simulink model "thread_id_calc"  (Simulink 7.7)
settings: Solver=ode45  StartTime=0.0  StopTime=100.0  RelTol=1e-3
undefined symbols (not defined in the file): xlipgetpartsetting
libraries: xbsIndex_r4 x50
settings Model: Creator=Andryc  LastModifiedBy=andryc

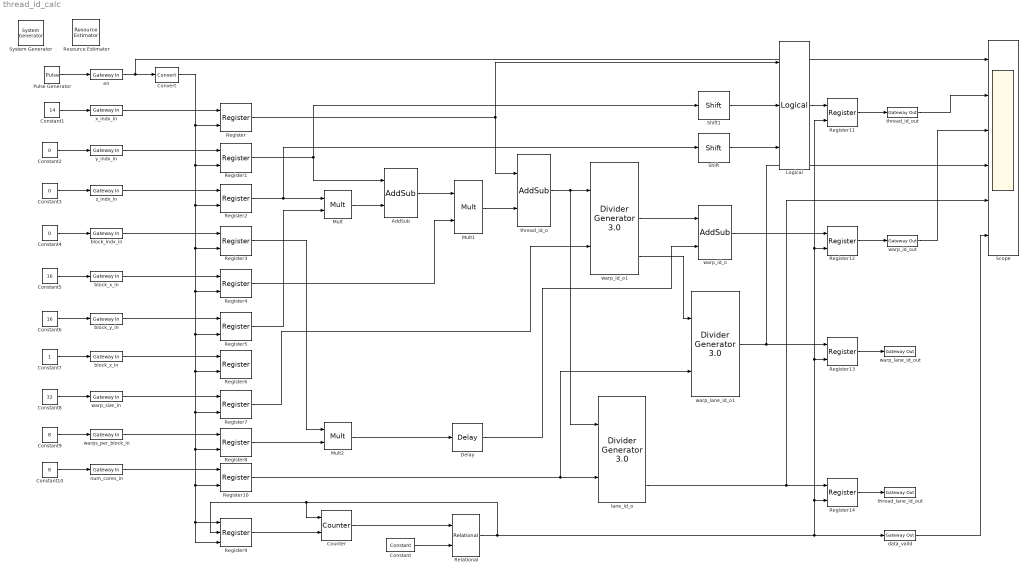
== system thread_id_calc ==
  " System Generator" : xbsIndex_r4/ System Generator  Tag=genX  SystemSampleTime=-1  xilinxfamily=virtex6  part=xc6vlx240t  speed=-2  package=ff1156  synthesis_tool=XST  clock_wrapper=Clock Enables  directory=./netlist  proj_type=Project Navigator  Synth_file=XST Defaults  Impl_file=ISE Defaults  testbench=on  simulink_period=1  sysclk_period=10  dcm_input_clock_period=10  incr_netlist=off  trim_vbits=Everywhere in SubSystem  dbl_ovrd=According to Block Masks  core_generation=According to Block Masks  run_coregen=off  deprecated_control=off  eval_field=0  block_type=sysgen
  AddSub : xbsIndex_r4/AddSub  mode=Addition  use_carryin=off  use_carryout=off  en=off  latency=0  precision=User Defined  arith_type=Unsigned  n_bits=32  bin_pt=0  quantization=Truncate  overflow=Saturate  dbl_ovrd=off  use_behavioral_HDL=off  hw_selection=Fabric  pipelined=off  block_type=addsub
  Constant : xbsIndex_r4/Constant  const=48  gui_display_data_type=Fixed-point  arith_type=Unsigned  n_bits=8  bin_pt=0  preci_type=Single  exp_width=8  frac_width=24  explicit_period=off  period=1  equ=P=C  opselect=C  inp2=PCIN>>17  opr=+  inp1=P  carry=CIN  dbl_ovrd=off  block_type=constant
  Constant1 : Constant  Value=14
  Constant10 : Constant  Value=8
  Constant2 : Constant  Value=0
  Constant3 : Constant  Value=0
  Constant4 : Constant  Value=0
  Constant5 : Constant  Value=16
  Constant6 : Constant  Value=16
  Constant7 : Constant
  Constant8 : Constant  Value=32
  Constant9 : Constant  Value=8
  Convert : xbsIndex_r4/Convert  gui_display_data_type=Boolean  arith_type=Boolean  n_bits=16  bin_pt=14  float_type=Single  exp_bits=8  fraction_bits=24  quantization=Truncate  overflow=Wrap  en=off  latency=0  dbl_ovrd=off  pipeline=off  block_type=convert
  Counter : xbsIndex_r4/Counter  cnt_type=Free Running  cnt_to=Inf  operation=Up  start_count=0  cnt_by_val=1  arith_type=Unsigned  n_bits=8  bin_pt=0  load_pin=off  rst=on  en=on  explicit_period=on  period=1  dbl_ovrd=off  use_behavioral_HDL=off  implementation=Fabric  block_type=counter
  Delay : xbsIndex_r4/Delay  rst=off  infoeditControl=Selection of Reset will increase slice count due to use of real FFs and instead of SRLs  en=off  latency=3  dbl_ovrd=off  reg_retiming=off  block_type=delay
  Logical : xbsIndex_r4/Logical  logical_function=OR  inputs=3  en=off  latency=0  precision=User Defined  arith_type=Unsigned  n_bits=32  bin_pt=0  align_bp=on  dbl_ovrd=off  block_type=logical
  Mult : xbsIndex_r4/Mult  precision=User Defined  arith_type=Unsigned  n_bits=32  bin_pt=0  quantization=Truncate  overflow=Saturate  en=off  latency=3  dbl_ovrd=off  use_behavioral_HDL=off  opt=Speed  use_embedded=on  optimum_pipeline=off  pipeline=on  use_rpm=on  placement_style=Triangular  block_type=mult
  Mult1 : xbsIndex_r4/Mult  precision=User Defined  arith_type=Unsigned  n_bits=32  bin_pt=0  quantization=Truncate  overflow=Saturate  en=off  latency=3  dbl_ovrd=off  use_behavioral_HDL=off  opt=Speed  use_embedded=on  optimum_pipeline=off  pipeline=on  use_rpm=on  placement_style=Triangular  block_type=mult
  Mult2 : xbsIndex_r4/Mult  precision=Full  arith_type="Signed  (2's comp)"  n_bits=16  bin_pt=14  quantization=Truncate  overflow=Wrap  en=off  latency=3  dbl_ovrd=off  use_behavioral_HDL=off  opt=Speed  use_embedded=on  optimum_pipeline=off  pipeline=on  use_rpm=on  placement_style=Triangular  block_type=mult
  Pulse Generator : DiscretePulseGenerator  Period=100  PhaseDelay=10
  Register{,1..8,10..14} (14 alike) : xbsIndex_r4/Register  init=0  rst=off  en=on  dbl_ovrd=off  block_type=register
  Register9 : xbsIndex_r4/Register  init=0  rst=on  en=on  dbl_ovrd=off  block_type=register
  Relational : xbsIndex_r4/Relational  mode=a=b  en=off  latency=0  dbl_ovrd=off  block_type=relational
  Resource Estimator : xbsIndex_r4/Resource Estimator  Tag=resEstTag  Slices=0  FFs=0  BRAMs=0  LUTs=0  IOBs=0  EBMs=0  TBUFs=0  xl_use_estimator_area=off  est_options=Estimate  block_type=resource_estimator
      settings: AttributesFormatString=Resource\nEstimator
  Scope : Scope  NumInputPorts=6
      settings: YMin=-5~-5~-5~-5~-5~-5  YMax=5~5~5~5~5~5
  Shift : xbsIndex_r4/Shift  shift_dir=Left  shift_bits=26  en=off  latency=0  precision=User Defined  arith_type=Unsigned  n_bits=32  bin_pt=0  quantization=Truncate  overflow=Saturate  dbl_ovrd=off  block_type=shift
  Shift1 : xbsIndex_r4/Shift  shift_dir=Left  shift_bits=16  en=off  latency=0  precision=User Defined  arith_type=Unsigned  n_bits=32  bin_pt=0  quantization=Truncate  overflow=Saturate  dbl_ovrd=off  block_type=shift
  block_indx_in : xbsIndex_r4/Gateway In  gui_display_data_type=Fixed-point  arith_type=Unsigned  n_bits=16  bin_pt=0  preci_type=Single  exp_width=8  frac_width=24  quantization=Truncate  overflow=Saturate  period=1  dbl_ovrd=off  timing_constraint=None  locs_specified=off  LOCs={}  inherit_from_input=off  UseAsADC=off  ADCChannel='1'  hdl_port=on  block_type=gatewayin
      settings: infoedit="Gateway in block.  Converts inputs of type Simulink integer, single, double and fixed point to  Xilinx fixed-point or floating-point data type.<br><br>Hardware notes:  In hardware these blocks become top level input ports."
  block_x_in : xbsIndex_r4/Gateway In  gui_display_data_type=Fixed-point  arith_type=Unsigned  n_bits=16  bin_pt=0  preci_type=Single  exp_width=8  frac_width=24  quantization=Truncate  overflow=Saturate  period=1  dbl_ovrd=off  timing_constraint=None  locs_specified=off  LOCs={}  inherit_from_input=off  UseAsADC=off  ADCChannel='1'  hdl_port=on  block_type=gatewayin
      settings: infoedit="Gateway in block.  Converts inputs of type Simulink integer, single, double and fixed point to  Xilinx fixed-point or floating-point data type.<br><br>Hardware notes:  In hardware these blocks become top level input ports."
  block_y_in : xbsIndex_r4/Gateway In  gui_display_data_type=Fixed-point  arith_type=Unsigned  n_bits=16  bin_pt=0  preci_type=Single  exp_width=8  frac_width=24  quantization=Truncate  overflow=Saturate  period=1  dbl_ovrd=off  timing_constraint=None  locs_specified=off  LOCs={}  inherit_from_input=off  UseAsADC=off  ADCChannel='1'  hdl_port=on  block_type=gatewayin
      settings: infoedit="Gateway in block.  Converts inputs of type Simulink integer, single, double and fixed point to  Xilinx fixed-point or floating-point data type.<br><br>Hardware notes:  In hardware these blocks become top level input ports."
  block_z_in : xbsIndex_r4/Gateway In  gui_display_data_type=Fixed-point  arith_type=Unsigned  n_bits=16  bin_pt=0  preci_type=Single  exp_width=8  frac_width=24  quantization=Truncate  overflow=Saturate  period=1  dbl_ovrd=off  timing_constraint=None  locs_specified=off  LOCs={}  inherit_from_input=off  UseAsADC=off  ADCChannel='1'  hdl_port=on  block_type=gatewayin
      settings: infoedit="Gateway in block.  Converts inputs of type Simulink integer, single, double and fixed point to  Xilinx fixed-point or floating-point data type.<br><br>Hardware notes:  In hardware these blocks become top level input ports."
  data_valid : xbsIndex_r4/Gateway Out  inherit_from_input=off  hdl_port=on  timing_constraint=None  locs_specified=off  LOCs={}  UseAsDAC=off  DACChannel='1'  block_type=gatewayout
      settings: infoedit="Gateway out block.  Converts Xilinx fixed-point or floating-point type inputs into ouputs of type Simulink integer, single, double, or fixed point.<br><br>Hardware notes:  In hardware these blocks become top level output ports or are discarded, depending on how they are configured."
  en : xbsIndex_r4/Gateway In  gui_display_data_type=Fixed-point  arith_type=Unsigned  n_bits=1  bin_pt=0  preci_type=Single  exp_width=8  frac_width=24  quantization=Truncate  overflow=Saturate  period=1  dbl_ovrd=off  timing_constraint=None  locs_specified=off  LOCs={}  inherit_from_input=off  UseAsADC=off  ADCChannel='1'  hdl_port=on  block_type=gatewayin
      settings: infoedit="Gateway in block.  Converts inputs of type Simulink integer, single, double and fixed point to  Xilinx fixed-point or floating-point data type.<br><br>Hardware notes:  In hardware these blocks become top level input ports."
  lane_id_o : xbsIndex_r4/Divider Generator 3.0   dividend_and_quotient_width=32  divisor_width=8  algorithm_type=Radix2  remainder_type=Remainder  fractional_width=16  clocks_per_division=1  divide_by_zero_detect=off  latency_configuration=Automatic  latency=20  ce=off  sclr=off  sclr_ce_priority=SCLR_overrides_CE  operand_sign=Signed  ip_name=Divider Generator  ip_version=3.0  dsptool_ready=true  wrapper_available=true  port_translation_map={ 'ce' => 'en', 'sclr' => 'rst' }  ipcore_fpga_part=xlipgetpartsetting(gcb, {'virtex4', 'xc4vsx35', '-10', 'ff668'})  ipcore_verbose=false  block_type=div_gen_v3_0
  num_cores_in : xbsIndex_r4/Gateway In  gui_display_data_type=Fixed-point  arith_type=Unsigned  n_bits=8  bin_pt=0  preci_type=Single  exp_width=8  frac_width=24  quantization=Truncate  overflow=Saturate  period=1  dbl_ovrd=off  timing_constraint=None  locs_specified=off  LOCs={}  inherit_from_input=off  UseAsADC=off  ADCChannel='1'  hdl_port=on  block_type=gatewayin
      settings: infoedit="Gateway in block.  Converts inputs of type Simulink integer, single, double and fixed point to  Xilinx fixed-point or floating-point data type.<br><br>Hardware notes:  In hardware these blocks become top level input ports."
  thread_id_o : xbsIndex_r4/AddSub  mode=Addition  use_carryin=off  use_carryout=off  en=off  latency=0  precision=User Defined  arith_type=Unsigned  n_bits=32  bin_pt=0  quantization=Truncate  overflow=Saturate  dbl_ovrd=off  use_behavioral_HDL=off  hw_selection=Fabric  pipelined=off  block_type=addsub
  thread_id_out : xbsIndex_r4/Gateway Out  inherit_from_input=off  hdl_port=on  timing_constraint=None  locs_specified=off  LOCs={}  UseAsDAC=off  DACChannel='1'  block_type=gatewayout
      settings: infoedit="Gateway out block.  Converts Xilinx fixed-point or floating-point type inputs into ouputs of type Simulink integer, single, double, or fixed point.<br><br>Hardware notes:  In hardware these blocks become top level output ports or are discarded, depending on how they are configured."
  thread_lane_id_out : xbsIndex_r4/Gateway Out  inherit_from_input=off  hdl_port=on  timing_constraint=None  locs_specified=off  LOCs={}  UseAsDAC=off  DACChannel='1'  block_type=gatewayout
      settings: infoedit="Gateway out block.  Converts Xilinx fixed-point or floating-point type inputs into ouputs of type Simulink integer, single, double, or fixed point.<br><br>Hardware notes:  In hardware these blocks become top level output ports or are discarded, depending on how they are configured."
  warp_id_o : xbsIndex_r4/AddSub  mode=Addition  use_carryin=off  use_carryout=off  en=off  latency=0  precision=User Defined  arith_type=Unsigned  n_bits=32  bin_pt=0  quantization=Truncate  overflow=Saturate  dbl_ovrd=off  use_behavioral_HDL=off  hw_selection=Fabric  pipelined=off  block_type=addsub
  warp_id_o1 : xbsIndex_r4/Divider Generator 3.0   dividend_and_quotient_width=32  divisor_width=6  algorithm_type=Radix2  remainder_type=Remainder  fractional_width=16  clocks_per_division=1  divide_by_zero_detect=off  latency_configuration=Automatic  latency=20  ce=off  sclr=off  sclr_ce_priority=SCLR_overrides_CE  operand_sign=Signed  ip_name=Divider Generator  ip_version=3.0  dsptool_ready=true  wrapper_available=true  port_translation_map={ 'ce' => 'en', 'sclr' => 'rst' }  ipcore_fpga_part=xlipgetpartsetting(gcb, {'virtex4', 'xc4vsx35', '-10', 'ff668'})  ipcore_verbose=false  block_type=div_gen_v3_0
  warp_id_out : xbsIndex_r4/Gateway Out  inherit_from_input=off  hdl_port=on  timing_constraint=None  locs_specified=off  LOCs={}  UseAsDAC=off  DACChannel='1'  block_type=gatewayout
      settings: infoedit="Gateway out block.  Converts Xilinx fixed-point or floating-point type inputs into ouputs of type Simulink integer, single, double, or fixed point.<br><br>Hardware notes:  In hardware these blocks become top level output ports or are discarded, depending on how they are configured."
  warp_lane_id_o1 : xbsIndex_r4/Divider Generator 3.0   dividend_and_quotient_width=6  divisor_width=8  algorithm_type=Radix2  remainder_type=Remainder  fractional_width=16  clocks_per_division=1  divide_by_zero_detect=off  latency_configuration=Automatic  latency=20  ce=off  sclr=off  sclr_ce_priority=SCLR_overrides_CE  operand_sign=Signed  ip_name=Divider Generator  ip_version=3.0  dsptool_ready=true  wrapper_available=true  port_translation_map={ 'ce' => 'en', 'sclr' => 'rst' }  ipcore_fpga_part=xlipgetpartsetting(gcb, {'virtex4', 'xc4vsx35', '-10', 'ff668'})  ipcore_verbose=false  block_type=div_gen_v3_0
  warp_lane_id_out : xbsIndex_r4/Gateway Out  inherit_from_input=off  hdl_port=on  timing_constraint=None  locs_specified=off  LOCs={}  UseAsDAC=off  DACChannel='1'  block_type=gatewayout
      settings: infoedit="Gateway out block.  Converts Xilinx fixed-point or floating-point type inputs into ouputs of type Simulink integer, single, double, or fixed point.<br><br>Hardware notes:  In hardware these blocks become top level output ports or are discarded, depending on how they are configured."
  warp_size_in : xbsIndex_r4/Gateway In  gui_display_data_type=Fixed-point  arith_type=Unsigned  n_bits=6  bin_pt=0  preci_type=Single  exp_width=8  frac_width=24  quantization=Truncate  overflow=Saturate  period=1  dbl_ovrd=off  timing_constraint=None  locs_specified=off  LOCs={}  inherit_from_input=off  UseAsADC=off  ADCChannel='1'  hdl_port=on  block_type=gatewayin
      settings: infoedit="Gateway in block.  Converts inputs of type Simulink integer, single, double and fixed point to  Xilinx fixed-point or floating-point data type.<br><br>Hardware notes:  In hardware these blocks become top level input ports."
  warps_per_block_in : xbsIndex_r4/Gateway In  gui_display_data_type=Fixed-point  arith_type=Unsigned  n_bits=6  bin_pt=0  preci_type=Single  exp_width=8  frac_width=24  quantization=Truncate  overflow=Saturate  period=1  dbl_ovrd=off  timing_constraint=None  locs_specified=off  LOCs={}  inherit_from_input=off  UseAsADC=off  ADCChannel='1'  hdl_port=on  block_type=gatewayin
      settings: infoedit="Gateway in block.  Converts inputs of type Simulink integer, single, double and fixed point to  Xilinx fixed-point or floating-point data type.<br><br>Hardware notes:  In hardware these blocks become top level input ports."
  x_indx_in : xbsIndex_r4/Gateway In  gui_display_data_type=Fixed-point  arith_type=Unsigned  n_bits=16  bin_pt=0  preci_type=Single  exp_width=8  frac_width=24  quantization=Truncate  overflow=Saturate  period=1  dbl_ovrd=off  timing_constraint=None  locs_specified=off  LOCs={}  inherit_from_input=off  UseAsADC=off  ADCChannel='1'  hdl_port=on  block_type=gatewayin
      settings: infoedit="Gateway in block.  Converts inputs of type Simulink integer, single, double and fixed point to  Xilinx fixed-point or floating-point data type.<br><br>Hardware notes:  In hardware these blocks become top level input ports."
  y_indx_in : xbsIndex_r4/Gateway In  gui_display_data_type=Fixed-point  arith_type=Unsigned  n_bits=16  bin_pt=0  preci_type=Single  exp_width=8  frac_width=24  quantization=Truncate  overflow=Saturate  period=1  dbl_ovrd=off  timing_constraint=None  locs_specified=off  LOCs={}  inherit_from_input=off  UseAsADC=off  ADCChannel='1'  hdl_port=on  block_type=gatewayin
      settings: infoedit="Gateway in block.  Converts inputs of type Simulink integer, single, double and fixed point to  Xilinx fixed-point or floating-point data type.<br><br>Hardware notes:  In hardware these blocks become top level input ports."
  z_indx_in : xbsIndex_r4/Gateway In  gui_display_data_type=Fixed-point  arith_type=Unsigned  n_bits=16  bin_pt=0  preci_type=Single  exp_width=8  frac_width=24  quantization=Truncate  overflow=Saturate  period=1  dbl_ovrd=off  timing_constraint=None  locs_specified=off  LOCs={}  inherit_from_input=off  UseAsADC=off  ADCChannel='1'  hdl_port=on  block_type=gatewayin
      settings: infoedit="Gateway in block.  Converts inputs of type Simulink integer, single, double and fixed point to  Xilinx fixed-point or floating-point data type.<br><br>Hardware notes:  In hardware these blocks become top level input ports."
  wires:
  x_indx_in/1 -> Register/1
  en/1 -> Convert/1, Scope/1
  Convert/1 -> Register/2, Register1/2, Register2/2, Register3/2, Register4/2, Register5/2, Register6/2, Register7/2, Register8/2, Register9/1, Register9/3, Register10/2
  y_indx_in/1 -> Register1/1
  z_indx_in/1 -> Register2/1
  block_indx_in/1 -> Register3/1
  block_x_in/1 -> Register4/1
  block_y_in/1 -> Register5/1
  warp_size_in/1 -> Register7/1
  block_z_in/1 -> Register6/1
  warps_per_block_in/1 -> Register8/1
  Register2/1 -> Mult/1, Shift/1
  Register5/1 -> Mult/2
  Mult/1 -> AddSub/2
  Register1/1 -> AddSub/1, Shift1/1
  AddSub/1 -> Mult1/1
  Register4/1 -> Mult1/2
  Mult1/1 -> thread_id_o/2
  Register/1 -> thread_id_o/1, Logical/1
  Register8/1 -> Mult2/2
  Register3/1 -> Mult2/1
  thread_id_o/1 -> warp_id_o1/1, lane_id_o/1
  Mult2/1 -> Delay/1
  Register7/1 -> warp_id_o1/2
  warp_id_o1/2 -> warp_id_o/1
  Delay/1 -> warp_id_o/2
  Shift/1 -> Logical/3
  Shift1/1 -> Logical/2
  Register9/1 -> Counter/2
  Counter/1 -> Relational/1
  Constant/1 -> Relational/2
  Relational/1 -> Counter/1, Register9/2, data_valid/1, Register14/2, Register13/2, Register12/2, Register11/2
  Pulse Generator/1 -> en/1
  Constant1/1 -> x_indx_in/1
  Constant2/1 -> y_indx_in/1
  Constant3/1 -> z_indx_in/1
  Constant4/1 -> block_indx_in/1
  Constant5/1 -> block_x_in/1
  Constant6/1 -> block_y_in/1
  Constant7/1 -> block_z_in/1
  Constant8/1 -> warp_size_in/1
  Constant9/1 -> warps_per_block_in/1
  num_cores_in/1 -> Register10/1
  Constant10/1 -> num_cores_in/1
  Register10/1 -> lane_id_o/2, warp_lane_id_o1/2
  Logical/1 -> Register11/1
  Register11/1 -> thread_id_out/1
  warp_id_o/1 -> Register12/1
  Register12/1 -> warp_id_out/1
  Register13/1 -> warp_lane_id_out/1
  lane_id_o/3 -> Register14/1, Scope/5
  Register14/1 -> thread_lane_id_out/1
  data_valid/1 -> Scope/6
  thread_id_out/1 -> Scope/2
  warp_lane_id_o1/2 -> Register13/1, Scope/4
  warp_id_o1/3 -> warp_lane_id_o1/1
  warp_id_out/1 -> Scope/3
